simulink library "tqd"  (R2021b)
settings: Solver=VariableStepAuto  StartTime=0.0  StopTime=10.0  RelTol=1e-3
undefined symbols (not defined in the file or in its folder): ATQD_APSDecReq_X_kph, ATQD_APSDecReq_Y_mps2, ATQD_APSDecReqCMD_X_kph, ATQD_APSDecReqTs_X_pct, ATQD_APSDecTimeGain_X_Deg, ATQD_APSDecTimeGain_Y_s, ATQD_APSReqLowSpd_X_Deg, ATQD_AutoHoldReleaseBPS_X_Deg, ATQD_AWDLoadTrqnsGain_X_kg, ATQD_AWDLoadTrqnsGain_Y_pct, ATQD_BOSEnBPSPosn_X_kph, ATQD_BOSMap_X_rpm, ATQD_BOSMap_Y_pct, ATQD_CreepBaseTqD_X_kph, ATQD_CreepBaseTqD_Y_Deg, ATQD_CreepBaseTqR_X_kph, ATQD_CreepBaseTqR_Y_Deg, ATQD_CreepBPSDisPosn_X_Deg, ATQD_CreepBPSDisPosnR_X_Deg, ATQD_CreepBPSEnPosn_X_Deg, ATQD_CreepBPSEnPosnR_X_Deg, ATQD_CreepDeltaTq_X_kph, ATQD_CreepIterm_X_kph, ATQD_CreepIterm_Y_kph, ATQD_CreepItermMaxLimit_X_pct, ATQD_CreepPreloadTime_X_kph, ATQD_CreepPreloadTq_X_kph, ATQD_CreepPreloadTq_Y_s, ATQD_CreepProtTq_X_Deg, ATQD_CreepPterm_X_kph, ATQD_ECOTqMapD_X_rpm, ATQD_ECOTqMapD_Y_pct, ATQD_EOPDTqMapDCon_X_rpm, ATQD_EOPDTqMapDCon_Y_Deg, ATQD_EstInitVehWeight_X_c, ATQD_LHMRollGenMapD_X_rpm, ATQD_LHMRollGenMapD_Y_rpm, ATQD_LHMTqMapD_X_rpm, ATQD_LHMTqMapD_Y_pct, ATQD_NL1TqMapD_X_rpm, ATQD_NL1TqMapD_Y_pct, ATQD_NOPDTqMapDCon_X_rpm, ATQD_NOPDTqMapDCon_Y_Deg, ATQD_NRMRrEDUSpRat_X_rpm, ATQD_NRMRrEDUSpRat_Y_Nm, ATQD_OPDHoldDownRelDelay_X_Deg, ATQD_OPDHoldEnSpd_X_Deg, ATQD_OPDHoldRelDetTime_X_Deg, ATQD_OPDHoldReleaseTq_X_Deg, ATQD_OrigPedTqLowLim_X_Deg, ATQD_OrigPedTqLowLim_Y_pct, ATQD_PedalMapClimbUpLim_X_rpm, ATQD_PedalMapClimbUpLim_Y_Deg, ATQD_PreLoadTq_X_s, ATQD_RollGenMapEL1_X_rpm, ATQD_RollGenMapEL1_Y_rpm, ATQD_SL1TqMapD_X_rpm, ATQD_SL1TqMapD_Y_pct, ATQD_SlideRegenTqGain_X_Gps, ATQD_SlideRegenTqGain_Y_pct ... (+444)
libraries: hcu_lib x70, simulink x61, tqr x1
(part 7 of 14)

== system tqd/TQD/TorqueDemand/TorqueModule/ExtTqFuncHandShaking ==
  VPMM_PwrSta_enum : Inport
  VTQD_MCUReady4Ext_flg : Inport  Port=2
  VINP_HVBattErr_flg : Inport  Port=3
  VINP_DCDCFaultSta_enum : Inport  Port=4
  VINP_EPBErrSta_enum : Inport  Port=5
  VINP_DrDoorSW_flg : Inport  Port=6
  VINP_PsDoorSW_flg : Inport  Port=7
  VINP_RRDoorSW_flg : Inport  Port=8
  VINP_RLDoorSW_flg : Inport  Port=9
  VINP_HoodSW_flg : Inport  Port=10
  VINP_TailgateSW_flg : Inport  Port=11
  Constant : Constant  Value=ENUM_POWERSTA_READY
  Constant1 : Constant  Value=KTQD_ExtTqAllow_flg_ovrdflg
  Constant10 : Constant  Value=TRUE
  Constant11 : Constant  Value=FALSE
  Constant12 : Constant  Value=ENUM_POWERSTA_READY
  Constant13 : Constant  Value=KTQD_ExtDoorAllow_flg_ovrdflg
  Constant14 : Constant  Value=KTQD_ExtDoorAllow_flg_ovrdval
  Constant2 : Constant  Value=ENUM_DCDCFAULTSTA_WORKING
  Constant3 : Constant  Value=KTQD_ExtTqAllow_flg_ovrdval
  Constant4 : Constant  Value=ENUM_DCDCFAULTSTA_WORKING
  Constant5 : Constant  Value=ENUM_EPBERROR_NORMAL
  Constant6 : Constant  Value=KTQD_ExtShftAllow_flg_ovrdflg
  Constant7 : Constant  Value=KTQD_ExtShftAllow_flg_ovrdval
  Constant8 : Constant  Value=TRUE
  Constant9 : Constant  Value=FALSE
  Equal{,1..4} (5 alike) : RelationalOperator  Operator===  OutDataTypeStr=boolean  RndMeth=Simplest
  LiuzgSwitch{1..5} (5 alike) : Switch  Criteria=u2 ~= 0
      settings: AttributesFormatString=<%<Criteria>>
  Logical Operator : Logic  Operator=NOT  AllPortsSameDT=off  OutDataTypeStr=boolean
  Logical Operator1 : Logic  Operator=NOT  AllPortsSameDT=off  OutDataTypeStr=boolean
  NOT{,1..5} (6 alike) : Logic  Operator=NOT  AllPortsSameDT=off  OutDataTypeStr=boolean
  OR : Logic  Inputs=4  AllPortsSameDT=off  OutDataTypeStr=boolean
  OR1 : Logic  Inputs=5  AllPortsSameDT=off  OutDataTypeStr=boolean
  OR2 : Logic  Inputs=6  AllPortsSameDT=off  OutDataTypeStr=boolean
  VTQD_ExternalTqAllow_flg : Outport
  VTQD_ExtShftAllow_flg : Outport  Port=2
  VTQD_ExtDoorAllow_flg : Outport  Port=3
  wires:
  Logical Operator/1 -> OR/2
  [VPMM_PwrSta_enum] -> Equal/1
  Constant/1 -> Equal/2
  VTQD_MCUReady4Ext_flg/1 -> [VTQD_MCUReady4Ext_flg]
  Constant2/1 -> Equal2/2
  [VINP_DCDCFaultSta_enum] -> Equal2/1
  Equal/1 -> OR/1
  [VTQD_MCUReady4Ext_flg] -> OR/4
  [VINP_HVBattErr_flg] -> Logical Operator/1
  Equal2/1 -> OR/3
  VINP_HVBattErr_flg/1 -> [VINP_HVBattErr_flg]
  VINP_DCDCFaultSta_enum/1 -> [VINP_DCDCFaultSta_enum]
  VPMM_PwrSta_enum/1 -> [VPMM_PwrSta_enum]
  LiuzgSwitch1/1 -> VTQD_ExternalTqAllow_flg/1  "VTQD_ExternalTqAllow_flg"
  Constant1/1 -> LiuzgSwitch1/2
  Constant3/1 -> LiuzgSwitch1/1
  VINP_EPBErrSta_enum/1 -> [VINP_EPBErrSta_enum]
  Constant5/1 -> Equal3/2
  LiuzgSwitch2/1 -> VTQD_ExtShftAllow_flg/1  "VTQD_ExtShftAllow_flg"
  Constant4/1 -> Equal1/2
  [VINP_HVBattErr_flg] -> Logical Operator1/1
  [VTQD_MCUReady4Ext_flg] -> OR1/4
  [VINP_EPBErrSta_enum] -> Equal3/1
  Equal1/1 -> OR1/2
  Equal3/1 -> OR1/1
  Logical Operator1/1 -> OR1/3
  [VINP_DCDCFaultSta_enum] -> Equal1/1
  Constant6/1 -> LiuzgSwitch2/2
  Constant7/1 -> LiuzgSwitch2/1
  OR1/1 -> LiuzgSwitch3/2
  LiuzgSwitch3/1 -> LiuzgSwitch2/3
  Constant8/1 -> LiuzgSwitch3/1
  Constant9/1 -> LiuzgSwitch3/3
  Constant11/1 -> LiuzgSwitch4/3
  Constant10/1 -> LiuzgSwitch4/1
  OR/1 -> LiuzgSwitch4/2
  LiuzgSwitch4/1 -> LiuzgSwitch1/3
  Constant12/1 -> Equal4/2
  [VPMM_PwrSta_enum] -> Equal4/1
  Equal4/1 -> OR1/5
  LiuzgSwitch5/1 -> VTQD_ExtDoorAllow_flg/1  "VTQD_ExtDoorAllow_flg"
  Constant14/1 -> LiuzgSwitch5/1
  Constant13/1 -> LiuzgSwitch5/2
  NOT5/1 -> OR2/6
  NOT4/1 -> OR2/5
  OR2/1 -> LiuzgSwitch5/3
  NOT2/1 -> OR2/3
  NOT/1 -> OR2/1
  NOT1/1 -> OR2/2
  NOT3/1 -> OR2/4
  [VINP_DrDoorSW_flg] -> NOT/1
  VINP_TailgateSW_flg/1 -> [VINP_TailgateSW_flg]
  VINP_RRDoorSW_flg/1 -> [VINP_RRDoorSW_flg]
  VINP_RLDoorSW_flg/1 -> [VINP_RLDoorSW_flg]
  VINP_HoodSW_flg/1 -> [VINP_HoodSW_flg]
  VINP_DrDoorSW_flg/1 -> [VINP_DrDoorSW_flg]
  VINP_PsDoorSW_flg/1 -> [VINP_PsDoorSW_flg]
  [VINP_PsDoorSW_flg] -> NOT1/1
  [VINP_RRDoorSW_flg] -> NOT2/1
  [VINP_RLDoorSW_flg] -> NOT3/1
  [VINP_HoodSW_flg] -> NOT4/1
  [VINP_TailgateSW_flg] -> NOT5/1

== system tqd/TQD/TorqueDemand/TorqueModule/OPD Hold ==
  task_time_s : Inport
  VTQD_RegenMode_enum : Inport  Port=2
  VTQD_GearActualPosn_enum : Inport  Port=3
  VTQD_VehActSpd_kph : Inport  Port=4
  VTQD_ActBPSPosn_pct : Inport  Port=5
  VVMC_ADASActive_flg : Inport  Port=6
  VVMC_CruzActive_flg : Inport  Port=7
  VTQD_ParkRequest_flg : Inport  Port=8
  VVMC_EstSlope_Deg : Inport  Port=9
  VVMC_LongAcc_Gps : Inport  Port=10
  VTQD_AntiBlockRrActDisTime_s : Inport  Port=11
  VTQD_RrAntiBlockAactive_flg : Inport  Port=12
  VTQD_AntiBlockFrActDisTime_s : Inport  Port=13
  VTQD_FrAntiBlockAactive_flg : Inport  Port=14
  VTQR_NoABSFEDUWhlTqReq_Nm : Inport  Port=15
  VTQR_NoABSREDUWhlTqReq_Nm : Inport  Port=16
  VINP_EPBSta_enum : Inport  Port=17
  VPMM_PwrSta_enum : Inport  Port=18
  VTQD_LowIdleAccPedal_flg : Inport  Port=19
  VTQD_ActAPSPosn_pct : Inport  Port=20
  VTQD_FrOPDHoldRelTqGain_Nm : Inport  Port=21
  VTQD_RrOPDHoldRelTqGain_Nm : Inport  Port=22
  Deceleration Calculation : Subsystem
  "OPDHold Request " : Subsystem
  Parking Requeest Backup : Subsystem
  Release Condition : Subsystem
  System Status : Subsystem
  VTQD_APSStaSys_enum : Outport
  VTQD_APSReq_enum : Outport  Port=2
  VTQD_APSDecReqA_flg : Outport  Port=3
  VTQD_APSDecReq_mps2 : Outport  Port=4
  VTQD_ActParkRequest_flg : Outport  Port=5
  VTQD_APSReqTimer_s : Outport  Port=6
  VTQD_OPDHoldEnRel_flg : Outport  Port=7
  VTQD_OPDHoldDelayForP_flg : Outport  Port=8
  VTQD_OPDHoldAllowPark_flg : Outport  Port=9
  VTQD_OPDHoldLamp_flg : Outport  Port=10
  VTQD_OPDHoldActRelTq_Nm : Outport  Port=11
  wires:
  VTQD_RegenMode_enum/1 -> [VTQD_RegenMode_enum]
  VTQD_GearActualPosn_enum/1 -> [VTQD_GearActualPosn_enum]
  VTQD_VehActSpd_kph/1 -> [VTQD_VehActSpd_kph]
  task_time_s/1 -> [task_time_s]
  [VTQD_APSStaSys_enum] -> VTQD_APSStaSys_enum/1
  [VTQD_APSReq_enum] -> VTQD_APSReq_enum/1
  [VTQD_APSDecReq_mps2] -> VTQD_APSDecReq_mps2/1
  [VTQD_APSDecReqA_flg] -> VTQD_APSDecReqA_flg/1
  VTQD_ActBPSPosn_pct/1 -> [VTQD_ActBPSPosn_pct]
  VVMC_ADASActive_flg/1 -> [VVMC_ADASActive_flg]
  VVMC_CruzActive_flg/1 -> [VVMC_CruzActive_flg]
  [VTQD_ActParkRequest_flg] -> VTQD_ActParkRequest_flg/1
  VTQD_ParkRequest_flg/1 -> [VTQD_ParkRequest_flg]
  VVMC_EstSlope_Deg/1 -> [VVMC_EstSlope_Deg]
  VVMC_LongAcc_Gps/1 -> [VVMC_LongAcc_Gps]
  VTQD_FrAntiBlockAactive_flg/1 -> [VTQD_FrAntiBlockAactive_flg]
  VTQD_AntiBlockFrActDisTime_s/1 -> [VTQD_AntiBlockFrActDisTime_s]
  VTQD_RrAntiBlockAactive_flg/1 -> [VTQD_RrAntiBlockAactive_flg]
  VTQD_AntiBlockRrActDisTime_s/1 -> [VTQD_AntiBlockRrActDisTime_s]
  VTQR_NoABSFEDUWhlTqReq_Nm/1 -> [VTQR_NoABSFEDUWhlTqReq_Nm]
  VTQR_NoABSREDUWhlTqReq_Nm/1 -> [VTQR_NoABSREDUWhlTqReq_Nm]
  VINP_EPBSta_enum/1 -> [VINP_EPBSta_enum]
  VPMM_PwrSta_enum/1 -> [VPMM_PwrSta_enum]
  [VTQD_OPDHoldDelayForP_flg] -> VTQD_OPDHoldDelayForP_flg/1
  [VTQD_APSReqTimer_s] -> VTQD_APSReqTimer_s/1
  [VTQD_OPDHoldEnRel_flg] -> VTQD_OPDHoldEnRel_flg/1
  [VTQD_AutoHoldRelease_flg] -> System Status/4(VTQD_AutiHoldRelease_flg)
  System Status/1(VTQD_APSStaSys_enum) -> [VTQD_APSStaSys_enum]
  [VTQD_ActBPSPosn_pct] -> Release Condition/5(VTQD_ActBPSPosn_pct)
  [VTQD_VehActSpd_kph] -> Release Condition/2(VTQD_VehActSpd_kph)
  Release Condition/1(VTQD_AutoHoldRelease_flg) -> [VTQD_AutoHoldRelease_flg]
  Release Condition/2(VTQD_OPDHoldEnRel_flg) -> [VTQD_OPDHoldEnRel_flg]
  System Status/2(VTQD_OPDHoldDelayForP_flg) -> [VTQD_OPDHoldDelayForP_flg]
  [VTQD_VehActSpd_kph] -> "OPDHold Request "/1(VTQD_VehActSpd_kph)
  [VTQD_APSStaSys_enum] -> "OPDHold Request "/2(VTQD_APSStaSys_enum)
  [VTQD_AutoHoldRelease_flg] -> "OPDHold Request "/3(VTQD_AutiHoldRelease_flg)
  [task_time_s] -> "OPDHold Request "/4(task_time_s)
  "OPDHold Request "/1(VTQD_APSReqTimer_s) -> [VTQD_APSReqTimer_s]
  "OPDHold Request "/2(VTQD_APSReq_enum) -> [VTQD_APSReq_enum]
  "OPDHold Request "/3(VTQD_APSDecReqA_flg) -> [VTQD_APSDecReqA_flg]
  [VTQD_VehActSpd_kph] -> Deceleration Calculation/1(VTQD_VehActSpd_kph)
  [VTQD_APSReqTimer_s] -> Deceleration Calculation/3(VTQD_APSReqTimer_s)
  [VVMC_EstSlope_Deg] -> Deceleration Calculation/4(VVMC_EstSlope_Deg)
  [VTQD_APSDecReqA_flg] -> Deceleration Calculation/5(VTQD_APSDecReqA_flg)
  Deceleration Calculation/1(VTQD_APSDecReq_mps2) -> [VTQD_APSDecReq_mps2]
  [VTQD_APSReq_enum] -> Parking Requeest Backup/1(VTQD_APSReq_enum)
  [VTQD_APSReqTimer_s] -> Parking Requeest Backup/2(VTQD_APSReqTimer_s)
  Parking Requeest Backup/1(VTQD_ActParkRequest_flg) -> [VTQD_ActParkRequest_flg]
  [VTQD_GearActualPosn_enum] -> System Status/1(VTQD_GearActualPosn_enum)
  [VINP_EPBSta_enum] -> System Status/2(VINP_EPBSta_enum)
  [VTQD_RegenMode_enum] -> System Status/3(VTQD_RegenMode_enum)
  [VTQD_AntiBlockRrActDisTime_s] -> System Status/5(VTQD_AntiBlockRrActDisTime_s)
  [VTQD_RrAntiBlockAactive_flg] -> System Status/6(VTQD_RrAntiBlockAactive_flg)
  [VTQD_ActBPSPosn_pct] -> System Status/7(VTQD_ActBPSPosn_pct)
  [VTQD_AntiBlockFrActDisTime_s] -> System Status/8(VTQD_AntiBlockFrActDisTime_s)
  [VTQD_FrAntiBlockAactive_flg] -> System Status/9(VTQD_FrAntiBlockAactive_flg)
  [VVMC_ADASActive_flg] -> System Status/10(VVMC_ADASActive_flg)
  [VPMM_PwrSta_enum] -> System Status/11(VPMM_PwrSta_enum)
  [VVMC_CruzActive_flg] -> System Status/12(VVMC_CruzActive_flg)
  [VTQD_VehActSpd_kph] -> System Status/13(VTQD_VehActSpd_kph)
  [VVMC_EstSlope_Deg] -> Release Condition/1(VVMC_EstSlope_Deg)
  [VTQR_NoABSFEDUWhlTqReq_Nm] -> Release Condition/3(VTQR_NoABSFEDUWhlTqReq_Nm)
  [VTQR_NoABSREDUWhlTqReq_Nm] -> Release Condition/4(VTQR_NoABSREDUWhlTqReq_Nm)
  [task_time_s] -> Release Condition/6(task_time_s)
  [VVMC_LongAcc_Gps] -> Deceleration Calculation/2(VVMC_LongAcc_Gps)
  [VTQD_ParkRequest_flg] -> Parking Requeest Backup/3(VTQD_ParkRequest_flg)
  [VTQD_AutoHoldRelease_flg] -> Deceleration Calculation/6(VTQD_AutiHoldRelease_flg)
  [VVMC_EstSlope_Deg] -> "OPDHold Request "/5(VVMC_EstSlope_Deg)
  [VTQD_APSReqTimer_s] -> Release Condition/7(VTQD_APSReqTimer_s)
  [VTQD_LowIdleAccPedal_flg] -> Release Condition/8(VTQD_LowIdleAccPedal_flg)
  VTQD_LowIdleAccPedal_flg/1 -> [VTQD_LowIdleAccPedal_flg]
  System Status/3(VTQD_OPDHoldRgnOn2Off_flg) -> [VTQD_OPDHoldRgnOn2Off_flg]
  [VTQD_OPDHoldRgnOn2Off_flg] -> Release Condition/9(VTQD_OPDHoldRgnOn2Off_flg)
  [task_time_s] -> Parking Requeest Backup/4(task_time_s)
  [VTQD_AutoHoldRelease_flg] -> Parking Requeest Backup/5(VTQD_AutiHoldRelease_flg)
  [task_time_s] -> Deceleration Calculation/7(task_time_s)
  [VTQD_ActAPSPosn_pct] -> Deceleration Calculation/8(VTQD_ActAPSPosn_pct)
  VTQD_ActAPSPosn_pct/1 -> [VTQD_ActAPSPosn_pct]
  Parking Requeest Backup/2(VTQD_OPDHoldAllowPark_flg) -> [VTQD_OPDHoldAllowPark_flg]
  [VTQD_OPDHoldAllowPark_flg] -> VTQD_OPDHoldAllowPark_flg/1
  [VTQD_ActAPSPosn_pct] -> Release Condition/10(VTQD_ActAPSPosn_pct)
  VTQD_RrOPDHoldRelTqGain_Nm/1 -> [VTQD_RrOPDHoldRelTqGain_Nm]
  VTQD_FrOPDHoldRelTqGain_Nm/1 -> [VTQD_FrOPDHoldRelTqGain_Nm]
  [VTQD_RrOPDHoldRelTqGain_Nm] -> Release Condition/12(VTQD_RrOPDHoldRelTqGain_Nm)
  [VTQD_FrOPDHoldRelTqGain_Nm] -> Release Condition/11(VTQD_FrOPDHoldRelTqGain_Nm)
  "OPDHold Request "/4(VTQD_OPDHoldLamp_flg) -> [VTQD_OPDHoldLamp_flg]
  [VTQD_OPDHoldLamp_flg] -> VTQD_OPDHoldLamp_flg/1
  [VTQD_OPDHoldActRelTq_Nm] -> VTQD_OPDHoldActRelTq_Nm/1
  Release Condition/3(VTQD_OPDHoldActRelTq_Nm) -> [VTQD_OPDHoldActRelTq_Nm]

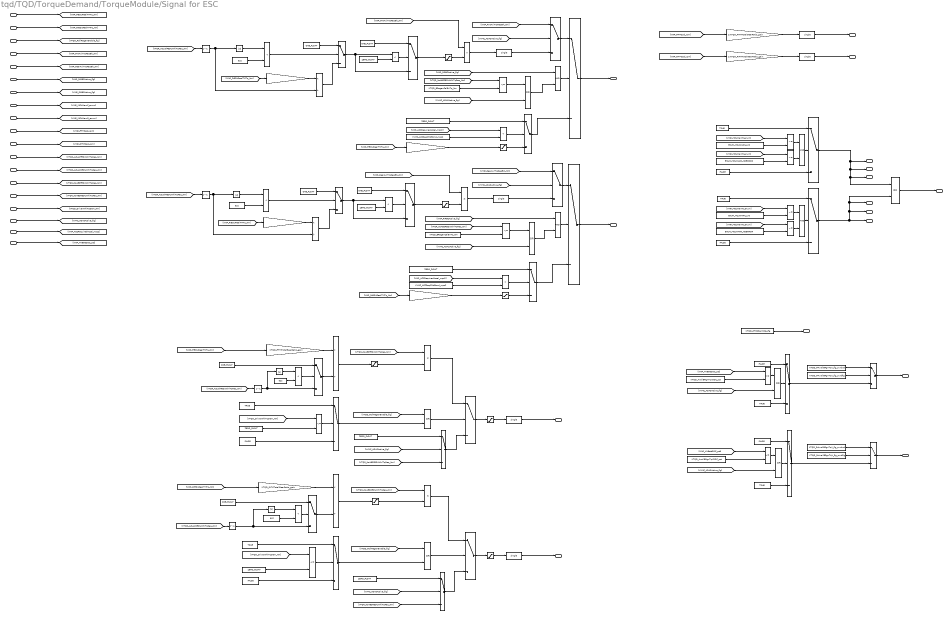
== system tqd/TQD/TorqueDemand/TorqueModule/Signal for ESC ==
  note: Front/Raer EDU actual torque (After Gearbox) calculation
  note: Front/Rear MCU error status signals
  note: Driving torque reduction permission status
  note: Front/Rear EDU speed (After Gearbox) calculation
  note: Front/Rear EDU rolling regen torque calculation
  VINP_FrEDURealTMTq_Nm : Inport
  VINP_RrEDURealTMTq_Nm : Inport  Port=2
  VTQD_RollRegenEnable_flg : Inport  Port=3
  VINP_FrntAxlTrqReqBrk_Nm : Inport  Port=4
  VINP_RearAxlTrqReqBrk_Nm : Inport  Port=5
  VINP_FrTMSpd_rpm : Inport  Port=6
  VINP_RrTMSpd_rpm : Inport  Port=7
  VINP_MCUWarnF_enum : Inport  Port=8
  VINP_MCUWarnR_enum : Inport  Port=9
  VINP_FrRBCActive_flg : Inport  Port=10
  VINP_RrRBCActive_flg : Inport  Port=11
  VTQR_ActualFEDUWhlTqReq_Nm : Inport  Port=12
  VTQR_ActualREDUWhlTqReq_Nm : Inport  Port=13
  VTQR_NoABSFEDUWhlTqReq_Nm : Inport  Port=14
  VTQR_NoABSREDUWhlTqReq_Nm : Inport  Port=15
  VTQD_DriverWhlTqDem_Nm : Inport  Port=16
  VVMC_ADASActive_flg : Inport  Port=17
  VINP_ACCRequiredAccel_mps2 : Inport  Port=18
  VINP_HVBattSOC_pct : Inport  Port=19
  AND1 : Logic  AllPortsSameDT=off  OutDataTypeStr=boolean
  AND2 : Logic  AllPortsSameDT=off  OutDataTypeStr=boolean
  Abs{,1..3} (4 alike) : Abs
  Constant1 : Constant  Value=KTQD_AvailBRgnTqVSOC_pct
  Constant{7,10,23,25,45,47..48,50} (8 alike) : Constant  Value=ZERO_FLOAT
  Constant{3,5,8,11,34,42} (6 alike) : Constant  Value=FALSE
  Constant{2,4,9,12,29,40} (6 alike) : Constant  Value=TRUE
  Constant13 : Constant  Value=KTQD_BRegenCalEnTq_Nm
  Constant{14,16,18,20} (4 alike) : Constant  Value=eps
  Constant15 : Constant  Value=KTQD_AvailBRgnTqVSOC_pct
  Constant{17,19,21..22,24,26} (6 alike) : Constant  Value=ONE_FLOAT
  Constant27 : Constant  Value=KTQD_FrAvailBRgnTqV_flg_ovrdflg
  Constant28 : Constant  Value=KTQD_FrAvailBRgnTqV_flg_ovrdval
  Constant30 : Constant  Value=KTQD_RrAvailBRgnTqV_flg_ovrdflg
  Constant31 : Constant  Value=KTQD_RrAvailBRgnTqV_flg_ovrdval
  Constant35 : Constant  Value=ENUM_MCUWARN_LV0
  Constant36 : Constant  Value=ENUM_MCUWARN_NOERROR
  Constant37 : Constant  Value=ENUM_MCUWARN_LV0
  Constant38 : Constant  Value=ENUM_MCUWARN_NOERROR
  Constant39 : Constant  Value=KTQD_BRegenCalEnTq_Nm
  Constant43 : Constant  Value=KVMC_ACCReqCMdBond_mps2
  Constant49 : Constant  Value=KVMC_ACCReqCMdBond_mps2
  Constant6 : Constant  Value=KTQD_PTCSPermSta_flg
  Data Type Conversion{1..3,5..7} (6 alike) : DataTypeConversion  OutDataTypeStr=single
  Delay{,1..3} (4 alike) : Delay  DelayLength=1
  Divide{,1,3,5} (4 alike) : Product  Inputs=*/
  Divide{2,4,6..7} (4 alike) : Product  Inputs=**
  Equal{,1..3,8..9} (6 alike) : RelationalOperator  Operator=<  OutDataTypeStr=boolean  RndMeth=Simplest
  Equal{4..7} (4 alike) : RelationalOperator  Operator=~=  OutDataTypeStr=boolean  RndMeth=Simplest
  Gain1 : Gain  Gain=1/KTQD_FrTMTotalGearRatio_gain
  Gain2 : Gain  Gain=1/KTQD_RrTMTotalGearRatio_gain
  Gain3 : Gain  Gain=KTQD_FrTMTotalGearRatio_gain
  Gain4 : Gain  Gain=KTQD_RrTMTotalGearRatio_gain
  Gain5 : Gain  Gain=KTQD_FrTMTotalGearRatio_gain
  Gain6 : Gain  Gain=KTQD_RrTMTotalGearRatio_gain
  Gain7 : Gain  Gain=KTQD_RrTMTotalGearRatio_gain
  Gain8 : Gain  Gain=KTQD_FrTMTotalGearRatio_gain
  Logical Operator : Logic  Operator=OR  AllPortsSameDT=off  OutDataTypeStr=boolean
  OR{,1,4..7} (6 alike) : Logic  Operator=OR  AllPortsSameDT=off  OutDataTypeStr=boolean
  OR2 : Logic  AllPortsSameDT=off  OutDataTypeStr=boolean
  OR3 : Logic  AllPortsSameDT=off  OutDataTypeStr=boolean
  Relational Operator{,1,4..5} (4 alike) : RelationalOperator  Operator=<=  OutDataTypeStr=boolean  RndMeth=Simplest
  Relational Operator2 : RelationalOperator  Operator=<  OutDataTypeStr=boolean  RndMeth=Simplest
  Relational Operator3 : RelationalOperator  Operator=<  OutDataTypeStr=boolean  RndMeth=Simplest
  Relational Operator6 : RelationalOperator  OutDataTypeStr=boolean  RndMeth=Simplest
  Relational Operator7 : RelationalOperator  OutDataTypeStr=boolean  RndMeth=Simplest
  Saturation : Saturate  UpperLimit=KTQD_FrBRgnCalUpLim_Nm  LowerLimit=KTQD_FrBRgnCalLowLim_Nm
      settings: AttributesFormatString=|
      | UpperLimit: %<UpperLimit>
      | LowerLimit: %<LowerLimit>
  Saturation1 : Saturate  UpperLimit=KTQD_RrBRgnCalUpLim_Nm  LowerLimit=KTQD_RrBRgnCalLowLim_Nm
      settings: AttributesFormatString=|
      | UpperLimit: %<UpperLimit>
      | LowerLimit: %<LowerLimit>
  Saturation2 : Saturate  UpperLimit=KTQD_RrEDURollRgnUpTq_Nm  LowerLimit=KTQD_RrEDURollRgnLowTq_Nm
      settings: AttributesFormatString=|
      | UpperLimit: %<UpperLimit>
      | LowerLimit: %<LowerLimit>
  Saturation3 : Saturate  UpperLimit=KTQD_FrEDURollRgnUpTq_Nm  LowerLimit=KTQD_FrEDURollRgnLowTq_Nm
  Saturation{4..7} (4 alike) : Saturate  UpperLimit=KTQD_TMTqDeviationUp_c  LowerLimit=KTQD_TMTqDeviationLow_c
      Saturation4 settings: AttributesFormatString=|
      | UpperLimit: %<UpperLimit>
      | LowerLimit: %<LowerLimit>
      Saturation5 settings: AttributesFormatString=|
      | UpperLimit: %<UpperLimit>
      | LowerLimit: %<LowerLimit>
      Saturation6 settings: LockScale=on
      Saturation6 settings: AttributesFormatString=|
      | UpperLimit: %<UpperLimit>
      | LowerLimit: %<LowerLimit>
      Saturation7 settings: AttributesFormatString=|
      | UpperLimit: %<UpperLimit>
      | LowerLimit: %<LowerLimit>
  Switch{,1..18,20..21,23} (22 alike) : Switch  Criteria=u2 ~= 0
  Switch19 : Switch  Criteria=u2 > Threshold
  Switch22 : Switch  Criteria=u2 > Threshold
  VTQD_FrEDUActTq_Nm : Outport
  VTQD_RrEDUActTq_Nm : Outport  Port=2
  VTQD_FrEDURolRgnTq_Nm : Outport  Port=3
  VTQD_RrEDURolRgnTq_Nm : Outport  Port=4
  VTQD_FrEDUSpd_rpm : Outport  Port=5
  VTQD_RrEDUSpd_rpm : Outport  Port=6
  VTQD_FrEDUSpdValid_flg : Outport  Port=7
  VTQD_FrEDUActTqValid_flg : Outport  Port=8
  VTQD_FrEDURolRgnTqValid_flg : Outport  Port=9
  VTQD_FrEDUAvailBrkRgnTqV_flg : Outport  Port=10
  VTQD_RrEDUSpdValid_flg : Outport  Port=11
  VTQD_RrEDUActTqValid_flg : Outport  Port=12
  VTQD_RrEDURolRgnTqValid_flg : Outport  Port=13
  VTQD_RrEDUAvailBrkRgnTqV_flg : Outport  Port=14
  VTQD_RgnAbnorSta_flg : Outport  Port=15
  VTQD_PTCSPermSta_flg : Outport  Port=16
  wires:
  Gain2/1 -> Data Type Conversion6/1
  Logical Operator/1 -> VTQD_RgnAbnorSta_flg/1  "VTQD_RgnAbnorSta_flg"
  Switch3/1 -> Logical Operator/1, VTQD_FrEDURolRgnTqValid_flg/1, VTQD_FrEDUActTqValid_flg/1, VTQD_FrEDUSpdValid_flg/1
  [VINP_FrTMSpd_rpm] -> Gain1/1
  Data Type Conversion2/1 -> VTQD_FrEDURolRgnTq_Nm/1  "VTQD_FrEDURolRgnTq_Nm"
  Data Type Conversion5/1 -> VTQD_FrEDUSpd_rpm/1  "VTQD_FrEDUSpd_rpm"
  Data Type Conversion3/1 -> VTQD_RrEDURolRgnTq_Nm/1  "VTQD_RrEDURolRgnTq_Nm"
  [VINP_RrTMSpd_rpm] -> Gain2/1
  Data Type Conversion6/1 -> VTQD_RrEDUSpd_rpm/1  "VTQD_RrEDUSpd_rpm"
  Switch2/1 -> VTQD_RrEDUActTqValid_flg/1, Logical Operator/2, VTQD_RrEDUSpdValid_flg/1, VTQD_RrEDURolRgnTqValid_flg/1
  Gain1/1 -> Data Type Conversion5/1
  Constant6/1 -> VTQD_PTCSPermSta_flg/1  "VTQD_PTCSPermSta_flg"
  Constant25/1 -> Relational Operator3/2
  Switch7/1 -> VTQD_FrEDUActTq_Nm/1  "VTQD_FrEDUActTq_Nm"
  [VINP_FrEDURealTMTq_Nm] -> Gain8/1
  Equal/1 -> Switch12/2
  [VINP_RrEDURealTMTq_Nm] -> Gain7/1
  Switch12/1 -> Switch14/3, Relational Operator2/1  "VTQD_FrTMTqDeviation_c"
  Constant21/1 -> Switch12/1
  [VTQR_ActualREDUWhlTqReq_Nm] -> Delay1/1
  Gain3/1 -> Divide/1
  Gain7/1 -> Saturation1/1
  Constant23/1 -> Relational Operator2/2
  [VINP_RrEDURealTMTq_Nm] -> Gain4/1
  Divide3/1 -> Switch13/3
  Divide/1 -> Switch12/3
  Delay/1 -> Divide/2, Abs3/1
  [VINP_FrEDURealTMTq_Nm] -> Gain3/1
  [VINP_RearAxlTrqReqBrk_Nm] -> Divide4/1
  [VINP_FrntAxlTrqReqBrk_Nm] -> Divide2/1
  Switch15/1 -> Saturation5/1  "VTQD_ActRrTMTqDeviation_c"
  [VTQR_ActualFEDUWhlTqReq_Nm] -> Delay/1
  Relational Operator2/1 -> Switch14/2
  Constant26/1 -> Switch15/1
  Switch13/1 -> Switch15/3, Relational Operator3/1  "VTQD_RrTMTqDeviation_c"
  Constant22/1 -> Switch13/1
  Saturation4/1 -> Divide2/2
  Switch10/1 -> VTQD_RrEDUActTq_Nm/1  "VTQD_RrEDUActTq_Nm"
  Gain8/1 -> Saturation/1
  Gain4/1 -> Divide3/1
  Relational Operator3/1 -> Switch15/2
  Constant24/1 -> Switch14/1
  Switch14/1 -> Saturation4/1  "VTQD_ActFrTMTqDeviation_c"
  Divide2/1 -> Data Type Conversion1/1  "VTQD_FrBRegenCal_Nm"
  Saturation5/1 -> Divide4/2
  Divide4/1 -> Data Type Conversion7/1  "VTQD_RrBRegenCal_Nm"
  Delay1/1 -> Abs2/1, Divide3/2
  Equal2/1 -> Switch13/2
  Gain5/1 -> Divide1/1
  Switch8/1 -> Divide1/2
  OR/1 -> Switch4/2
  Switch5/1 -> OR/2  "VTQD_FrWhlTqDemNeg_flg"
  Delay2/1 -> Abs/1, Switch8/3
  [VTQR_ActualFEDUWhlTqReq_Nm] -> Delay2/1
  Constant17/1 -> Switch8/1
  [VTQD_DriverWhlTqDem_Nm] -> Relational Operator/1
  Constant9/1 -> Switch5/1
  Equal1/1 -> Switch8/2
  [VTQD_RollRegenEnable_flg] -> OR/1
  [VINP_FrEDURealTMTq_Nm] -> Gain5/1
  Switch4/1 -> Saturation3/1
  Constant7/1 -> Relational Operator/2
  Divide6/1 -> Switch4/1  "VTQD_FrARegenCal_Nm"
  [VTQR_NoABSFEDUWhlTqReq_Nm] -> Divide6/1
  Relational Operator/1 -> Switch5/2
  Constant8/1 -> Switch5/3
  Saturation3/1 -> Data Type Conversion2/1
  Saturation6/1 -> Divide6/2
  Divide1/1 -> Saturation6/1
  Constant10/1 -> Relational Operator1/2
  Gain6/1 -> Divide5/1
  Delay3/1 -> Abs1/1, Switch11/3
  [VTQR_ActualREDUWhlTqReq_Nm] -> Delay3/1
  Switch6/1 -> Saturation2/1
  Saturation2/1 -> Data Type Conversion3/1
  OR1/1 -> Switch6/2
  [VINP_RrEDURealTMTq_Nm] -> Gain6/1
  [VTQD_RollRegenEnable_flg] -> OR1/1
  Constant12/1 -> Switch9/1
  Switch9/1 -> OR1/2  "VTQD_RrWhlTqDemNeg_flg"
  [VTQD_DriverWhlTqDem_Nm] -> Relational Operator1/1
  [VTQR_NoABSREDUWhlTqReq_Nm] -> Divide7/1
  Equal3/1 -> Switch11/2
  Saturation7/1 -> Divide7/2
  Divide7/1 -> Switch6/1  "VTQD_RrARegenCal_Nm"
  Switch11/1 -> Divide5/2
  Constant19/1 -> Switch11/1
  Divide5/1 -> Saturation7/1
  Constant11/1 -> Switch9/3
  Relational Operator1/1 -> Switch9/2
  Constant30/1 -> Switch17/2
  Constant31/1 -> Switch17/1
  Constant28/1 -> Switch16/1
  Constant27/1 -> Switch16/2
  Switch16/1 -> VTQD_FrEDUAvailBrkRgnTqV_flg/1
  Switch17/1 -> VTQD_RrEDUAvailBrkRgnTqV_flg/1
  Constant2/1 -> Switch2/1
  [VINP_MCUWarnF_enum] -> Equal5/1
  OR2/1 -> Switch3/2
  Equal5/1 -> OR2/2
  Constant36/1 -> Equal5/2
  Constant35/1 -> Equal4/2
  [VINP_MCUWarnF_enum] -> Equal4/1
  Constant5/1 -> Switch3/3
  Equal6/1 -> OR3/1
  Equal4/1 -> OR2/1
  [VINP_MCUWarnR_enum] -> Equal6/1
  [VINP_MCUWarnR_enum] -> Equal7/1
  Constant4/1 -> Switch3/1
  Constant37/1 -> Equal6/2
  Constant38/1 -> Equal7/2
  Constant3/1 -> Switch2/3
  OR3/1 -> Switch2/2
  Equal7/1 -> OR3/2
  VINP_FrEDURealTMTq_Nm/1 -> [VINP_FrEDURealTMTq_Nm]
  VINP_RrEDURealTMTq_Nm/1 -> [VINP_RrEDURealTMTq_Nm]
  VTQD_RollRegenEnable_flg/1 -> [VTQD_RollRegenEnable_flg]
  VINP_FrntAxlTrqReqBrk_Nm/1 -> [VINP_FrntAxlTrqReqBrk_Nm]
  VINP_MCUWarnF_enum/1 -> [VINP_MCUWarnF_enum]
  VTQR_ActualFEDUWhlTqReq_Nm/1 -> [VTQR_ActualFEDUWhlTqReq_Nm]
  VTQR_ActualREDUWhlTqReq_Nm/1 -> [VTQR_ActualREDUWhlTqReq_Nm]
  VTQR_NoABSFEDUWhlTqReq_Nm/1 -> [VTQR_NoABSFEDUWhlTqReq_Nm]
  VTQR_NoABSREDUWhlTqReq_Nm/1 -> [VTQR_NoABSREDUWhlTqReq_Nm]
  VTQD_DriverWhlTqDem_Nm/1 -> [VTQD_DriverWhlTqDem_Nm]
  VINP_FrRBCActive_flg/1 -> [VINP_FrRBCActive_flg]
  VINP_MCUWarnR_enum/1 -> [VINP_MCUWarnR_enum]
  VINP_FrTMSpd_rpm/1 -> [VINP_FrTMSpd_rpm]
  VINP_RrTMSpd_rpm/1 -> [VINP_RrTMSpd_rpm]
  VINP_RearAxlTrqReqBrk_Nm/1 -> [VINP_RearAxlTrqReqBrk_Nm]
  VINP_RrRBCActive_flg/1 -> [VINP_RrRBCActive_flg]
  AND1/1 -> Switch10/2
  Constant13/1 -> Relational Operator4/2
  [VINP_FrRBCActive_flg] -> AND2/1
  [VTQR_NoABSFEDUWhlTqReq_Nm] -> Relational Operator4/1
  AND2/1 -> Switch7/2
  Constant39/1 -> Relational Operator5/2
  [VTQR_NoABSREDUWhlTqReq_Nm] -> Relational Operator5/1
  [VINP_RrRBCActive_flg] -> AND1/1
  Data Type Conversion1/1 -> Switch1/3
  Switch1/1 -> Switch7/1
  VVMC_ADASActive_flg/1 -> [VVMC_ADASActive_flg]
  [VVMC_ADASActive_flg] -> Switch1/2
  [VINP_FrntAxlTrqReqBrk_Nm] -> Switch1/1
  Data Type Conversion7/1 -> Switch18/3
  Switch18/1 -> Switch10/1
  [VINP_RearAxlTrqReqBrk_Nm] -> Switch18/1
  Constant34/1 -> Switch20/1
  Constant40/1 -> Switch21/3
  Constant29/1 -> Switch20/3
  Constant42/1 -> Switch21/1
  Switch21/1 -> Switch17/3
  Switch20/1 -> Switch16/3
  [VVMC_ADASActive_flg] -> OR5/2
  Relational Operator4/1 -> OR5/1
  OR5/1 -> AND2/2
  [VVMC_ADASActive_flg] -> OR4/2
  Relational Operator5/1 -> OR4/1
  OR4/1 -> AND1/2
  [VTQR_NoABSFEDUWhlTqReq_Nm] -> Switch19/3
  Constant47/1 -> Switch19/1
  Switch19/1 -> Switch4/3
  [VVMC_ADASActive_flg] -> Switch19/2
  Switch22/1 -> Switch6/3
  Constant45/1 -> Switch22/1
  [VTQR_NoABSREDUWhlTqReq_Nm] -> Switch22/3
  [VVMC_ADASActive_flg] -> Switch22/2
  Saturation/1 -> Switch/3
  Constant43/1 -> Equal8/2
  Equal8/1 -> Switch/2
  VINP_ACCRequiredAccel_mps2/1 -> [VINP_ACCRequiredAccel_mps2]
  [VINP_ACCRequiredAccel_mps2] -> Equal8/1
  Switch/1 -> Switch7/3
  Constant48/1 -> Switch/1
  Constant50/1 -> Switch23/1
  Equal9/1 -> Switch23/2
  [VINP_ACCRequiredAccel_mps2] -> Equal9/1
  Constant49/1 -> Equal9/2
  Saturation1/1 -> Switch23/3
  Switch23/1 -> Switch10/3
  Constant14/1 -> Equal/2
  Constant16/1 -> Equal2/2
  Constant18/1 -> Equal1/2
  Constant20/1 -> Equal3/2
  [VVMC_ADASActive_flg] -> Switch18/2
  [VINP_HVBattSOC_pct] -> Relational Operator6/1
  Constant1/1 -> Relational Operator6/2
  OR6/1 -> Switch21/2
  Relational Operator6/1 -> OR6/1
  [VVMC_ADASActive_flg] -> OR6/2
  Constant15/1 -> Relational Operator7/2
  Relational Operator7/1 -> OR7/1
  [VINP_HVBattSOC_pct] -> Relational Operator7/1
  OR7/1 -> Switch20/2
  [VVMC_ADASActive_flg] -> OR7/2
  VINP_HVBattSOC_pct/1 -> [VINP_HVBattSOC_pct]
  Abs/1 -> Equal1/1
  Abs1/1 -> Equal3/1
  Abs2/1 -> Equal2/1
  Abs3/1 -> Equal/1

== system tqd/TQD/TorqueDemand/TorqueModule/Signals for BCM ==
  VTQD_ARegenActive_flg : Inport
  VINP_LongAccel_Gps : Inport  Port=2
  Constant : Constant  Value=KVMC_GravityValue_mps2
  Logical Operator : Logic  AllPortsSameDT=off  OutDataTypeStr=boolean
  Product : Product
  Relay1 : Relay  OnSwitchValue=KTQD_RegBrkLPOff_c  OffSwitchValue=KTQD_RegBrkLPOn_c  OnOutputValue=0  OffOutputValue=1
      settings: AttributesFormatString=|
      | ON: %<OnSwitchValue>
      | OFF: %<OffSwitchValue>
  VTQD_ReBrakeLPReq_flg : Outport
  wires:
  VINP_LongAccel_Gps/1 -> [VINP_LongAccel_Gps]
  Relay1/1 -> Logical Operator/2
  Logical Operator/1 -> VTQD_ReBrakeLPReq_flg/1  "VTQD_ReBrakeLPReq_flg"
  Constant/1 -> Product/1
  [VTQD_ARegenActive_flg] -> Logical Operator/1
  Product/1 -> Relay1/1
  [VINP_LongAccel_Gps] -> Product/2
  VTQD_ARegenActive_flg/1 -> [VTQD_ARegenActive_flg]

== system tqd/TQD/TorqueDemand/TorqueModule/Signals for MCU ==
  Constant : Constant  Value=KTQD_FrIdcMin_A
  Constant1 : Constant  Value=KTQD_FrIdcMax_A
  Constant2 : Constant  Value=KTQD_FrUdcMax_V
  Constant3 : Constant  Value=KTQD_FrUdcMin_V
  Constant4 : Constant  Value=KTQD_RrIdcMin_A
  Constant5 : Constant  Value=KTQD_RrIdcMax_A
  Constant6 : Constant  Value=KTQD_RrUdcMax_V
  Constant7 : Constant  Value=KTQD_RrUdcMin_V
  VTQD_FrIdcMin_A : Outport
  VTQD_FrIdcMax_A : Outport  Port=2
  VTQD_FrUdcMin_V : Outport  Port=3
  VTQD_FrUdcMax_V : Outport  Port=4
  VTQD_RrIdcMin_A : Outport  Port=5
  VTQD_RrIdcMax_A : Outport  Port=6
  VTQD_RrUdcMin_V : Outport  Port=7
  VTQD_RrUdcMax_V : Outport  Port=8
  wires:
  Constant4/1 -> VTQD_RrIdcMin_A/1  "VTQD_RrIdcMin_A"
  Constant6/1 -> VTQD_RrUdcMax_V/1  "VTQD_RrUdcMax_V"
  Constant5/1 -> VTQD_RrIdcMax_A/1  "VTQD_RrIdcMax_A"
  Constant7/1 -> VTQD_RrUdcMin_V/1  "VTQD_RrUdcMin_V"
  Constant2/1 -> VTQD_FrUdcMax_V/1  "VTQD_FrUdcMax_V"
  Constant3/1 -> VTQD_FrUdcMin_V/1  "VTQD_FrUdcMin_V"
  Constant1/1 -> VTQD_FrIdcMax_A/1  "VTQD_FrIdcMax_A"
  Constant/1 -> VTQD_FrIdcMin_A/1  "VTQD_FrIdcMin_A"

== system tqd/TQD/TorqueDemand/TorqueModule/TqCoordination ==
  note: Wheel torque coordination
  VTQD_GearActualPosn_enum : Inport
  VVMC_ADASActive_flg : Inport  Port=2
  VVMC_ADASWhlTqReq_Nm : Inport  Port=3
  VVMC_CruzActive_flg : Inport  Port=4
  VVMC_CruzWhlTqReq_Nm : Inport  Port=5
  VVMC_MSAActive_flg : Inport  Port=6
  VVMC_MSAWhlTqReq_Nm : Inport  Port=7
  VVMC_APSActive_flg : Inport  Port=8
  VTQD_DriverWhlTqDem_Nm : Inport  Port=9
  VINP_ADASForceIdle_flg : Inport  Port=10
  VTQD_PreLoadHold_flg : Inport  Port=11
  Constant1 : Constant  Value=ENUM_GEARACTUALPOSN_R
  Constant2 : Constant  Value=ENUM_GEARACTUALPOSN_D
  Coordinate_ADAS : Subsystem  AncestorBlock=tqd162/TQD/TorqueDemand/TorqueModule/TqCoordination/Coordinate_FrADAS  TreatAsAtomicUnit=on
  Coordinate_ADASForceIdle : Subsystem  TreatAsAtomicUnit=on
  Coordinate_APS : Subsystem  TreatAsAtomicUnit=on
  Coordinate_Cruise : Subsystem  AncestorBlock=tqd162/TQD/TorqueDemand/TorqueModule/TqCoordination/Coordinate_FrCruise  TreatAsAtomicUnit=on
  Coordinate_DirverPedal : Subsystem  AncestorBlock=tqd/TQD/TorqueDemand/TorqueModule/TqCoordination/If Action Subsystem4  TreatAsAtomicUnit=on
  Coordinate_MSA : Subsystem  AncestorBlock=tqd162/TQD/TorqueDemand/TorqueModule/TqCoordination/Coordinate_FrMSA  TreatAsAtomicUnit=on
  Coordinate_NoSuitbleGear_flg : Subsystem  TreatAsAtomicUnit=on
  Data Type Conversion2 : DataTypeConversion  OutDataTypeStr=uint8
  Equal1 : RelationalOperator  Operator===  OutDataTypeStr=boolean  RndMeth=Simplest
  Equal4 : RelationalOperator  Operator===  OutDataTypeStr=boolean  RndMeth=Simplest
  If : If  NumInputs=6  IfExpression=u1 ~= 0  ElseIfExpressions=u2 ~= 0, u3 ~= 0, u4 ~= 0, u5 ~= 0, u6 ~= 0
  Merge4 : Merge  Inputs=7
  Merge5 : Merge  Inputs=7
  NOT1 : Logic  Operator=NOT  AllPortsSameDT=off  OutDataTypeStr=boolean
  OR1 : Logic  Operator=OR  AllPortsSameDT=off  OutDataTypeStr=boolean
  VTQD_CoordTqDem_Nm : Outport
  VTQD_TqSource_enum : Outport  Port=2
  wires:
  Coordinate_ADASForceIdle/2(VTQD_ADASForceIdle_enum) -> [VTQD_ADASForceIdle_enum]
  Coordinate_ADASForceIdle/1(VTQD_ADASForceIdleReq_Nm) -> [VTQD_ADASForceIdleReq_Nm]
  Coordinate_DirverPedal/2(VTQD_TqSourceInternal_enum) -> [VTQD_TqSourceInternal_enum]
  Coordinate_DirverPedal/1(VTQD_DriverWhlTqReq_Nm) -> [VTQD_DriverWhlTqReq_Nm]
  [VTQD_NoSuitbleGear_flg] -> If/1
  Equal4/1 -> OR1/1
  Constant2/1 -> Equal4/1
  VTQD_GearActualPosn_enum/1 -> [VTQD_GearActualPosn_enum]
  Coordinate_NoSuitbleGear_flg/1(VTQD_GearNoSuitReq_Nm) -> [VTQD_GearNoSuitReq_Nm]
  OR1/1 -> NOT1/1
  Coordinate_APS/1(VTQD_APSWhlTqReq_Nm) -> [VTQD_APSWhlTqReq_Nm]
  Coordinate_APS/2(VTQD_TqSourceAPS_enum) -> [VTQD_TqSourceAPS_enum]
  NOT1/1 -> [VTQD_NoSuitbleGear_flg]  "VTQD_NoSuitbleGear_flg"
  [VTQD_GearActualPosn_enum] -> Equal4/2, Equal1/1
  Equal1/1 -> OR1/2
  Coordinate_NoSuitbleGear_flg/2(VTQD_TqSourceGearNoSuit_enum) -> [VTQD_TqSourceGearNoSuit_enum]
  Constant1/1 -> Equal1/2
  VVMC_ADASActive_flg/1 -> [VVMC_ADASActive_flg]
  VTQD_DriverWhlTqDem_Nm/1 -> [VTQD_DriverWhlTqDem_Nm]
  VVMC_ADASWhlTqReq_Nm/1 -> [VVMC_ADASWhlTqReq_Nm]
  VINP_ADASForceIdle_flg/1 -> [VINP_ADASForceIdle_flg]
  VVMC_MSAActive_flg/1 -> [VVMC_MSAActive_flg]
  VVMC_CruzWhlTqReq_Nm/1 -> [VVMC_CruzWhlTqReq_Nm]
  VVMC_MSAWhlTqReq_Nm/1 -> [VVMC_MSAWhlTqReq_Nm]
  VVMC_APSActive_flg/1 -> [VVMC_APSActive_flg]
  VVMC_CruzActive_flg/1 -> [VVMC_CruzActive_flg]
  VTQD_PreLoadHold_flg/1 -> [VTQD_PreLoadHold_flg]
  If/1 -> Coordinate_NoSuitbleGear_flg/Action
  Coordinate_ADAS/1(VTQD_ADASWhlTqReq_Nm) -> [VTQD_ADASWhlTqReq_Nm]
  Coordinate_ADAS/2(VTQD_TqSourceADAS_enum) -> [VTQD_TqSourceADAS_enum]
  [VTQD_PreLoadHold_flg] -> Coordinate_ADAS/2(VTQD_PreLoadHold_flg)
  Coordinate_Cruise/2(VTQD_TqSourceCruz_enum) -> [VTQD_TqSourceCruz_enum]
  Coordinate_MSA/2(VTQD_TqSourceMSA_enum) -> [VTQD_TqSourceMSA_enum]
  Coordinate_Cruise/1(VTQD_CruzWhlTqReq_Nm) -> [VTQD_CruzWhlTqReq_Nm]
  Coordinate_MSA/1(VTQD_MSAWhlTqReq_Nm) -> [VTQD_MSAWhlTqReq_Nm]
  [VINP_ADASForceIdle_flg] -> If/2
  [VVMC_ADASActive_flg] -> If/3
  [VVMC_CruzActive_flg] -> If/4
  [VVMC_MSAActive_flg] -> If/5
  [VVMC_APSActive_flg] -> If/6
  If/2 -> Coordinate_ADASForceIdle/Action
  If/3 -> Coordinate_ADAS/Action
  [VVMC_ADASWhlTqReq_Nm] -> Coordinate_ADAS/1(VVMC_ADASWhlTqReq_Nm)
  [VTQD_DriverWhlTqDem_Nm] -> Coordinate_ADAS/3(VTQD_DriverWhlTqDem_Nm)
  If/4 -> Coordinate_Cruise/Action
  [VVMC_CruzWhlTqReq_Nm] -> Coordinate_Cruise/1(VVMC_CruzWhlTqReq_Nm)
  If/5 -> Coordinate_MSA/Action
  [VVMC_MSAWhlTqReq_Nm] -> Coordinate_MSA/1(VVMC_MSAWhlTqReq_Nm)
  If/6 -> Coordinate_APS/Action
  [VTQD_DriverWhlTqDem_Nm] -> Coordinate_APS/1(VTQD_DriverWhlTqDem_Nm)
  If/7 -> Coordinate_DirverPedal/Action
  [VTQD_DriverWhlTqDem_Nm] -> Coordinate_DirverPedal/1(VTQD_DriverWhlTqDem_Nm)
  [VTQD_ADASForceIdle_enum] -> Merge5/7
  [VTQD_DriverWhlTqReq_Nm] -> Merge4/6
  [VTQD_MSAWhlTqReq_Nm] -> Merge4/4
  [VTQD_GearNoSuitReq_Nm] -> Merge4/1
  [VTQD_TqSourceCruz_enum] -> Merge5/3
  [VTQD_TqSourceInternal_enum] -> Merge5/6
  [VTQD_TqSourceMSA_enum] -> Merge5/4
  [VTQD_TqSourceAPS_enum] -> Merge5/5
  Merge4/1 -> VTQD_CoordTqDem_Nm/1  "VTQD_CoordTqDem_Nm"
  [VTQD_ADASForceIdleReq_Nm] -> Merge4/7
  Merge5/1 -> Data Type Conversion2/1
  [VTQD_TqSourceGearNoSuit_enum] -> Merge5/1
  Data Type Conversion2/1 -> VTQD_TqSource_enum/1  "VTQD_TqSource_enum"
  [VTQD_ADASWhlTqReq_Nm] -> Merge4/2
  [VTQD_APSWhlTqReq_Nm] -> Merge4/5
  [VTQD_CruzWhlTqReq_Nm] -> Merge4/3
  [VTQD_TqSourceADAS_enum] -> Merge5/2

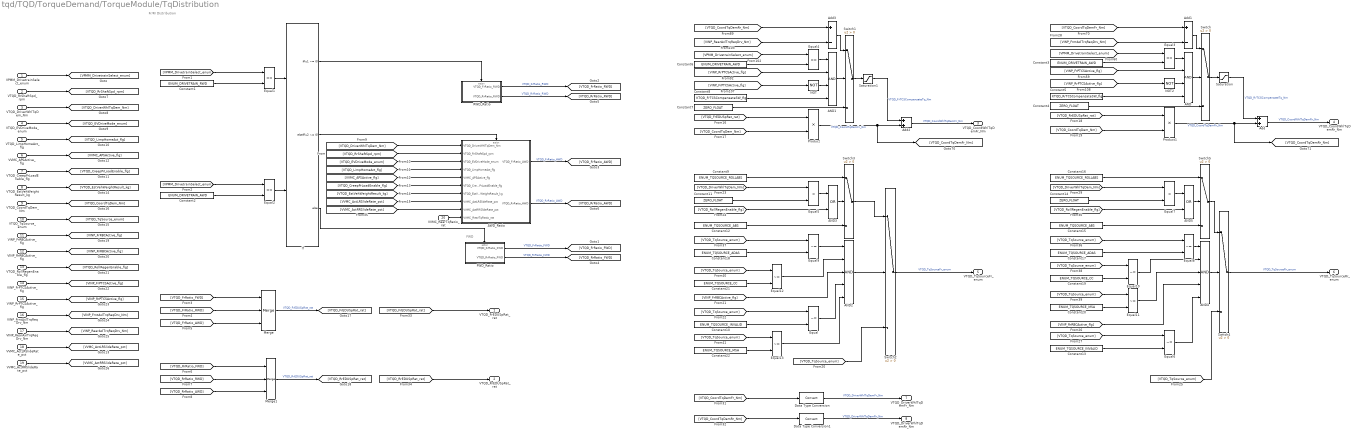
== system tqd/TQD/TorqueDemand/TorqueModule/TqDistribution ==
  note: Fr/Rr Distribution
  note: FWD
  VPMM_DrivetrainSelect_enum : Inport
  VTQD_RrShaftSpd_rpm : Inport  Port=2
  VTQD_DriverWhlTqDem_Nm : Inport  Port=3
  VTQD_EVDriveMode_enum : Inport  Port=4
  VTQD_LimpHomeAct_flg : Inport  Port=5
  VVMC_APSActive_flg : Inport  Port=6
  VTQD_CreepPrLoadEnable_flg : Inport  Port=7
  VTQD_EstVehWeightResult_kg : Inport  Port=8
  VTQD_CoordTqDem_Nm : Inport  Port=9
  VTQD_TqSource_enum : Inport  Port=10
  VINP_FrRBCActive_flg : Inport  Port=11
  VINP_RrRBCActive_flg : Inport  Port=12
  VTQD_RollRegenEnable_flg : Inport  Port=13
  VINP_FrPTCSActive_flg : Inport  Port=14
  VINP_RrPTCSActive_flg : Inport  Port=15
  VINP_FrntAxlTrqReqDrv_Nm : Inport  Port=16
  VINP_RearAxlTrqReqDrv_Nm : Inport  Port=17
  VVMC_ActLRSlideRate_pct : Inport  Port=18
  VVMC_ActRRSlideRate_pct : Inport  Port=19
  VVMC_RearTqRatio_rat : Inport  Port=20
  AND : Logic  Inputs=4  AllPortsSameDT=off  OutDataTypeStr=boolean
  AND1 : Logic  Inputs=4  AllPortsSameDT=off  OutDataTypeStr=boolean
  AND2 : Logic  Inputs=5  AllPortsSameDT=off  OutDataTypeStr=boolean
  AND3 : Logic  Operator=OR  AllPortsSameDT=off  OutDataTypeStr=boolean
  AND4 : Logic  Inputs=5  AllPortsSameDT=off  OutDataTypeStr=boolean
  AND5 : Logic  Operator=OR  AllPortsSameDT=off  OutDataTypeStr=boolean
  AWD_Ratio : Subsystem  TreatAsAtomicUnit=on
  Add : Sum
  Add1 : Sum  Inputs=+-
  Add2 : Sum
  Add3 : Sum  Inputs=+-
  Constant1 : Constant  Value=ENUM_DRIVETRAIN_RWD  VectorParams1D=off  SampleTime=-1
  Constant10 : Constant  Value=ENUM_TQSOURCE_INVALID  VectorParams1D=off  SampleTime=-1
  Constant{4,7,11,14} (4 alike) : Constant  Value=ZERO_FLOAT  VectorParams1D=off  SampleTime=-1
  Constant12 : Constant  Value=ENUM_TQSOURCE_ABS  VectorParams1D=off  SampleTime=-1
  Constant13 : Constant  Value=ENUM_TQSOURCE_INVALID  VectorParams1D=off  SampleTime=-1
  Constant15 : Constant  Value=ENUM_TQSOURCE_ABS  VectorParams1D=off  SampleTime=-1
  Constant16 : Constant  Value=ENUM_TQSOURCE_ROLLABS  VectorParams1D=off  SampleTime=-1
  Constant17 : Constant  Value=ENUM_TQSOURCE_ADAS  VectorParams1D=off  SampleTime=-1
  Constant18 : Constant  Value=ENUM_TQSOURCE_ADAS  VectorParams1D=off  SampleTime=-1
  Constant19 : Constant  Value=ENUM_TQSOURCE_CC  SampleTime=-1
  Constant2 : Constant  Value=ENUM_DRIVETRAIN_AWD  VectorParams1D=off  SampleTime=-1
  Constant20 : Constant  Value=ENUM_TQSOURCE_MSA  SampleTime=-1
  Constant21 : Constant  Value=ENUM_TQSOURCE_CC  SampleTime=-1
  Constant22 : Constant  Value=ENUM_TQSOURCE_MSA  SampleTime=-1
  Constant3 : Constant  Value=ENUM_DRIVETRAIN_AWD  VectorParams1D=off  SampleTime=-1
  Constant5 : Constant  Value=KTQD_RrTCSCompensateSW_flg  VectorParams1D=off  SampleTime=-1
  Constant6 : Constant  Value=ENUM_DRIVETRAIN_AWD  VectorParams1D=off  SampleTime=-1
  Constant8 : Constant  Value=KTQD_FrTCSCompensateSW_flg  VectorParams1D=off  SampleTime=-1
  Constant9 : Constant  Value=ENUM_TQSOURCE_ROLLABS  VectorParams1D=off  SampleTime=-1
  Data Type Conversion : DataTypeConversion
  Data Type Conversion1 : DataTypeConversion
  Equal{,6,8..13} (8 alike) : RelationalOperator  Operator=~=  OutDataTypeStr=boolean  RndMeth=Simplest
  Equal{1..4} (4 alike) : RelationalOperator  Operator===  OutDataTypeStr=boolean  RndMeth=Simplest
  Equal5 : RelationalOperator  Operator=<  OutDataTypeStr=boolean  RndMeth=Simplest
  Equal7 : RelationalOperator  Operator=<  OutDataTypeStr=boolean  RndMeth=Simplest
  FWD_Ratio : Subsystem  TreatAsAtomicUnit=on
  If : If  NumInputs=2  IfExpression=u1 ~= 0  ElseIfExpressions=u2 ~= 0
  Merge : Merge  Inputs=3
  Merge1 : Merge  Inputs=3
  NOT : Logic  Operator=NOT  AllPortsSameDT=off  OutDataTypeStr=boolean
  NOT2 : Logic  Operator=NOT  AllPortsSameDT=off  OutDataTypeStr=boolean
  Product : Product
  Product1 : Product
  RWD_Ratio : Subsystem  TreatAsAtomicUnit=on
  Saturation : Saturate  UpperLimit=KTQD_TCSCompUpLimit_Nm  LowerLimit=ZERO_FLOAT
  Saturation1 : Saturate  UpperLimit=KTQD_TCSCompUpLimit_Nm  LowerLimit=ZERO_FLOAT
  Switch{,1..5} (6 alike) : Switch  Criteria=u2 > Threshold
  VTQD_FrEDUSpRat_rat : Outport
  VTQD_RrEDUSpRat_rat : Outport  Port=2
  VTQD_CoordWhlTqDemFr_Nm : Outport  Port=3
  VTQD_CoordWhlTqDemRr_Nm : Outport  Port=4
  VTQD_TqSourceFr_enum : Outport  Port=5
  VTQD_TqSourceRr_enum : Outport  Port=6
  VTQD_DriverWhlTqDemFr_Nm : Outport  Port=7
  VTQD_DriverWhlTqDemRr_Nm : Outport  Port=8
  wires:
  VPMM_DrivetrainSelect_enum/1 -> [VPMM_DrivetrainSelect_enum]
  Constant1/1 -> Equal1/2
  [VPMM_DrivetrainSelect_enum] -> Equal1/1
  [VPMM_DrivetrainSelect_enum] -> Equal2/1
  Constant2/1 -> Equal2/2
  Equal2/1 -> If/2
  FWD_Ratio/1(VTQD_FrRatio_FWD) -> [VTQD_FrRatio_FWD]  "VTQD_FrRatio_FWD"
  FWD_Ratio/2(VTQD_RrRatio_FWD) -> [VTQD_RrRatio_FWD]  "VTQD_RrRatio_FWD"
  RWD_Ratio/1(VTQD_FrRatio_RWD) -> [VTQD_FrRatio_RWD]  "VTQD_FrRatio_RWD"
  RWD_Ratio/2(VTQD_RrRatio_RWD) -> [VTQD_RrRatio_RWD]  "VTQD_RrRatio_RWD"
  [VTQD_FrRatio_FWD] -> Merge/1
  [VTQD_FrRatio_RWD] -> Merge/2
  [VTQD_FrRatio_AWD] -> Merge/3
  [VTQD_RrRatio_FWD] -> Merge1/1
  [VTQD_RrRatio_RWD] -> Merge1/2
  [VTQD_RrRatio_AWD] -> Merge1/3
  AWD_Ratio/1(VTQD_FrRatio_AWD) -> [VTQD_FrRatio_AWD]  "VTQD_FrRatio_AWD"
  AWD_Ratio/2(VTQD_RrRatio_AWD) -> [VTQD_RrRatio_AWD]  "VTQD_RrRatio_AWD"
  Equal1/1 -> If/1
  If/1 -> RWD_Ratio/Action
  If/2 -> AWD_Ratio/Action
  If/3 -> FWD_Ratio/Action
  VTQD_RrShaftSpd_rpm/1 -> [VTQD_RrShaftSpd_rpm]
  VTQD_DriverWhlTqDem_Nm/1 -> [VTQD_DriverWhlTqDem_Nm]
  [VTQD_DriverWhlTqDem_Nm] -> AWD_Ratio/1(VTQD_DriverWhlTqDem_Nm)
  [VTQD_RrShaftSpd_rpm] -> AWD_Ratio/2(VTQD_RrShaftSpd_rpm)
  VTQD_EVDriveMode_enum/1 -> [VTQD_EVDriveMode_enum]
  [VTQD_EVDriveMode_enum] -> AWD_Ratio/3(VTQD_EVDriveMode_enum)
  VTQD_LimpHomeAct_flg/1 -> [VTQD_LimpHomeAct_flg]
  [VTQD_LimpHomeAct_flg] -> AWD_Ratio/4(VTQD_LimpHomeAct_flg)
  VTQD_CreepPrLoadEnable_flg/1 -> [VTQD_CreepPrLoadEnable_flg]
  [VTQD_CreepPrLoadEnable_flg] -> AWD_Ratio/6(VTQD_CreepPrLoadEnable_flg)
  [VVMC_APSActive_flg] -> AWD_Ratio/5(VVMC_APSActive_flg)
  VVMC_APSActive_flg/1 -> [VVMC_APSActive_flg]
  VTQD_EstVehWeightResult_kg/1 -> [VTQD_EstVehWeightResult_kg]
  [VTQD_EstVehWeightResult_kg] -> AWD_Ratio/7(VTQD_EstVehWeightResult_kg)
  Merge/1 -> [VTQD_FrEDUSpRat_rat]  "VTQD_FrEDUSpRat_rat"
  Merge1/1 -> [VTQD_RrEDUSpRat_rat]  "VTQD_RrEDUSpRat_rat"
  [VTQD_FrEDUSpRat_rat] -> VTQD_FrEDUSpRat_rat/1
  [VTQD_RrEDUSpRat_rat] -> VTQD_RrEDUSpRat_rat/1
  Switch3/1 -> Switch2/1
  AND4/1 -> Switch4/2
  Add2/1 -> VTQD_CoordWhlTqDemFr_Nm/1  "VTQD_CoordWhlTqDemFr_Nm"
  [VTQD_CoordTqDemFr_Nm] -> Data Type Conversion/1
  Equal5/1 -> AND3/1
  Data Type Conversion/1 -> VTQD_DriverWhlTqDemFr_Nm/1  "VTQD_DriverWhlTqDemFr_Nm"
  [VINP_FrPTCSActive_flg] -> AND/2
  Equal7/1 -> AND5/1
  [VTQD_DriverWhlTqDem_Nm] -> Equal5/1
  [VTQD_TqSource_enum] -> Switch4/3
  [VTQD_RollRegenEnable_flg] -> AND5/2
  [VTQD_RollRegenEnable_flg] -> AND3/2
  Constant6/1 -> Equal4/2
  Constant12/1 -> Switch3/3
  Switch5/1 -> Switch4/1
  Constant9/1 -> Switch3/1
  AND/1 -> Switch/2
  AND1/1 -> Switch1/2
  [VTQD_DriverWhlTqDem_Nm] -> Equal7/1
  Constant14/1 -> Equal7/2
  AND5/1 -> Switch5/2
  Constant10/1 -> Equal/2
  [VTQD_CoordTqDemRr_Nm] -> Data Type Conversion1/1
  [VINP_RearAxlTrqReqDrv_Nm] -> Add3/2
  Constant16/1 -> Switch5/1
  Constant4/1 -> Switch/3
  Switch4/1 -> VTQD_TqSourceRr_enum/1  "VTQD_TqSourceRr_enum"
  Constant11/1 -> Equal5/2
  [VINP_RrPTCSActive_flg] -> NOT2/1
  AND3/1 -> Switch3/2
  [VINP_FrntAxlTrqReqDrv_Nm] -> Add1/2
  Product1/1 -> [VTQD_CoordTqDemRr_Nm], Add/2  "VTQD_CoordTqDemRr_Nm"
  [VTQD_TqSource_enum] -> Switch2/3
  Data Type Conversion1/1 -> VTQD_DriverWhlTqDemRr_Nm/1  "VTQD_DriverWhlTqDemRr_Nm"
  [VTQD_RrEDUSpRat_rat] -> Product1/1
  [VTQD_TqSource_enum] -> Equal6/1
  [VTQD_CoordTqDem_Nm] -> Product/2
  [VPMM_DrivetrainSelect_enum] -> Equal4/1
  [VTQD_CoordTqDem_Nm] -> Product1/2
  Constant5/1 -> AND/4
  Constant13/1 -> Equal6/2
  NOT/1 -> AND1/3
  Add/1 -> VTQD_CoordWhlTqDemRr_Nm/1  "VTQD_CoordWhlTqDemRr_Nm"
  Equal4/1 -> AND1/1
  [VPMM_DrivetrainSelect_enum] -> Equal3/1
  [VINP_FrPTCSActive_flg] -> NOT/1
  [VTQD_CoordTqDemRr_Nm] -> Add3/1
  Equal3/1 -> AND/1
  [VTQD_TqSource_enum] -> Equal/1
  Constant3/1 -> Equal3/2
  Constant8/1 -> AND1/4
  Switch/1 -> Saturation/1
  Add3/1 -> Switch1/1
  Switch1/1 -> Saturation1/1
  Add1/1 -> Switch/1
  Constant7/1 -> Switch1/3
  Constant15/1 -> Switch5/3
  Saturation1/1 -> Add2/1  "VTQD_FrTCSCompensateTq_Nm"
  NOT2/1 -> AND/3
  [VINP_RrPTCSActive_flg] -> AND1/2
  Switch2/1 -> VTQD_TqSourceFr_enum/1  "VTQD_TqSourceFr_enum"
  Product/1 -> [VTQD_CoordTqDemFr_Nm], Add2/2  "VTQD_CoordTqDemFr_Nm"
  [VTQD_CoordTqDemFr_Nm] -> Add1/1
  [VTQD_FrEDUSpRat_rat] -> Product/1
  Saturation/1 -> Add/1  "VTQD_RrTCSCompensateTq_Nm"
  VINP_RrPTCSActive_flg/1 -> [VINP_RrPTCSActive_flg]
  VINP_RearAxlTrqReqDrv_Nm/1 -> [VINP_RearAxlTrqReqDrv_Nm]
  VTQD_CoordTqDem_Nm/1 -> [VTQD_CoordTqDem_Nm]
  VINP_FrntAxlTrqReqDrv_Nm/1 -> [VINP_FrntAxlTrqReqDrv_Nm]
  VTQD_RollRegenEnable_flg/1 -> [VTQD_RollRegenEnable_flg]
  VINP_RrRBCActive_flg/1 -> [VINP_RrRBCActive_flg]
  VTQD_TqSource_enum/1 -> [VTQD_TqSource_enum]
  VINP_FrRBCActive_flg/1 -> [VINP_FrRBCActive_flg]
  VINP_FrPTCSActive_flg/1 -> [VINP_FrPTCSActive_flg]
  VVMC_ActLRSlideRate_pct/1 -> [VVMC_ActLRSlideRate_pct]
  VVMC_ActRRSlideRate_pct/1 -> [VVMC_ActRRSlideRate_pct]
  [VVMC_ActLRSlideRate_pct] -> AWD_Ratio/8(VVMC_ActLRSlideRate_pct)
  [VVMC_ActRRSlideRate_pct] -> AWD_Ratio/9(VVMC_ActRRSlideRate_pct)
  Constant17/1 -> Equal8/2
  [VTQD_TqSource_enum] -> Equal8/1
  Equal6/1 -> AND4/5
  Equal8/1 -> AND4/1
  [VINP_RrRBCActive_flg] -> AND4/4
  AND2/1 -> Switch2/2
  [VINP_FrRBCActive_flg] -> AND2/3
  [VTQD_TqSource_enum] -> Equal9/1
  Constant18/1 -> Equal9/2
  Equal/1 -> AND2/4
  Equal9/1 -> AND2/1
  [VTQD_TqSource_enum] -> Equal10/1
  Constant19/1 -> Equal10/2
  Equal10/1 -> AND4/2
  Constant20/1 -> Equal11/2
  [VTQD_TqSource_enum] -> Equal11/1
  Equal11/1 -> AND4/3
  [VTQD_TqSource_enum] -> Equal13/1
  Constant22/1 -> Equal13/2
  Constant21/1 -> Equal12/2
  [VTQD_TqSource_enum] -> Equal12/1
  Equal12/1 -> AND2/2
  Equal13/1 -> AND2/5
  VVMC_RearTqRatio_rat/1 -> AWD_Ratio/10(VVMC_RearTqRatio_rat)
